simulink model "PowerGenSim_Attitude"  (R2024b)
settings: Solver=ode3  StartTime=0.0  StopTime=sat.T  FixedStep=10  MaxStep=113.53623125513354  RelTol=1e-3
values from neighbouring files (symbols this model uses):
  Re = 6378e03    (= 6378000)    [PowerGenSim_Params.m]
undefined symbols (not defined in the file or in its folder): sat
libraries: sharedtransform x4, vrlib x4, slpidlib x4, matrix_library x2, aerolibutil x1, sharedutil x1, aerolibsatdyn x1, simulink_extras x1
settings Model: Creator=Ameya  LastModifiedBy=Ameya

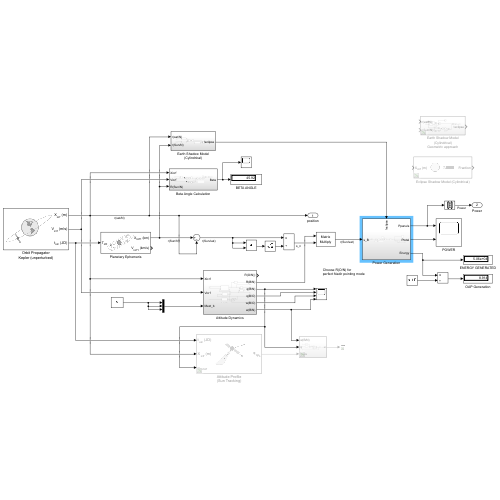
[thumbnail: Simulink's stored preview of the top-level diagram]
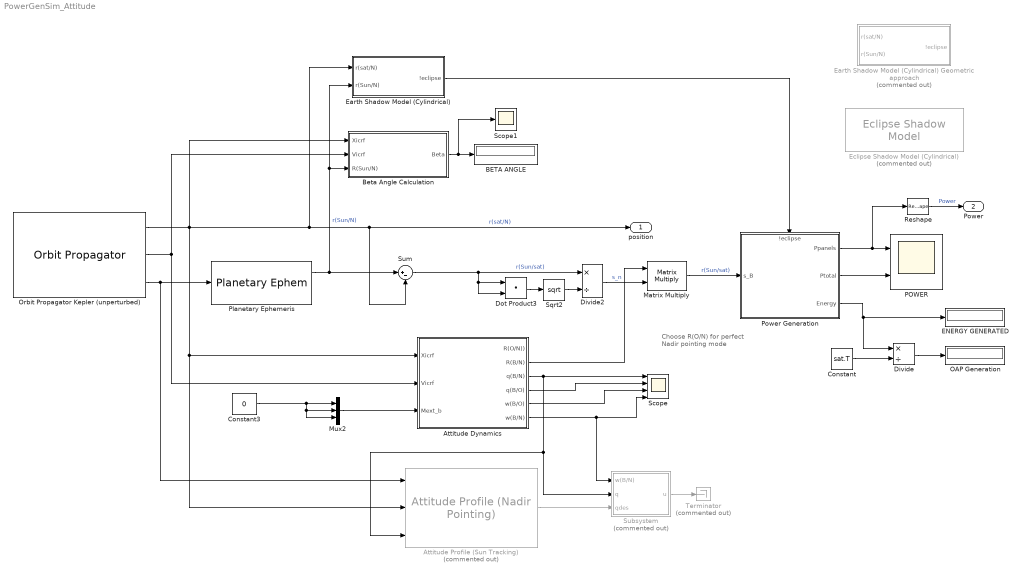
== system PowerGenSim_Attitude ==
  note: Choose R(O/N) for
      | perfect Nadir pointing mode
  Attitude Dynamics : Subsystem
  Attitude Profile (Sun Tracking) : aerolibsatdyn/Attitude Profile (Nadir Pointing)  Commented=on  outputError=on  outputFinalAttitude=off  portFrame=ICRF  pointingMode=Point at celestial body  celestialTarget=Sun  tunablePointing=off  primaryAlignmentSrc=Dialog  primaryAlignment=[0 0 1]  secondaryAlignmentSrc=Dialog  secondaryAlignment=[1 0 0]  constraintFrame=ICRF  primaryConstraintSrc=Dialog  primaryConstraint=[1 0 0]  secondaryConstraintSrc=Dialog  secondaryConstraint=[0 1 0]
      settings: LibrarySourceBlock=|
      | aerolibsatdyn/Attitude Profile
      | (Sun Tracking)
  BETA ANGLE : Display
  Beta Angle Calculation : Subsystem
  Constant : Constant  Value=sat.T
  Constant3 : Constant  Value=0
  Divide : Product  Inputs=*/
  Divide2 : Product  Inputs=*/
  Dot Product3 : DotProduct  OutDataTypeStr=Inherit: Inherit via internal rule
  ENERGY GENERATED : Display
  Earth Shadow Model (Cylindrical) : Subsystem
  Earth Shadow Model (Cylindrical) Geometric approach : Subsystem  Commented=on
  Eclipse Shadow Model (Cylindrical) : EclipseShadowModel  Commented=on  shadowModel=Cylindrical  startDate=initialTimeJD  includeMoon=off  useEphemerisDateRange=off
  Matrix Multiply : Product  Multiplication=Matrix(*)
  Mux2 : Mux  Inputs=3
  OAP Generation : Display
  Orbit Propagator Kepler (unperturbed) : OrbitPropagator  startDate=initialTimeJD  semiMajorAxis=sat.a  eccentricity=sat.e  inclination=sat.i  raan=sat.RAAN  argPeriapsis=sat.w  trueAnomaly=sat.f  inertialPosition=[3649700.0 3308200.0 -4676600.0]  inertialVelocity=[-2750.8 6666.4 2573.4]  fixedPosition=[-4142689.0 -2676864.7 -4669861.6]  fixedVelocity=[1452.7 -6720.7 2568.1]  customR=3396200  customMu=4.305e13  customJ2=1.0826269e-03  customOmega=4.06125949e-3
  POWER : Scope  NumInputPorts=2
  Planetary Ephemeris : PlanetaryEphem  target=Sun
  Power Generation : Subsystem
      settings: PortSchema="{\"entries\":[{\"content\":{\"sides\":[{\"content\":{\"connectorIds\":[\"In1\"]},\"type\":\"ConnectorPlacement.EquallySpacedRectSide\",\"uuid\":\"8d446733-69e8-48a0-ae35-006265559fdb\"},{\"content\":{\"connectorIds\":[\"Out1\",\"Out2\",\"Out3\"],\"side\":\"RIGHT\"},\"type\":\"ConnectorPlacement.EquallySpacedRectSide\",\"uuid\":\"081b3f49-1ee9-4aa1-bea1-61239cdc4507\"},{\"content\":{\"connectorIds\":[\"In2\"],\"side\":\"TOP\"},\"type\":\"ConnectorPlacement.EquallySpacedRectSide\",\"uuid\":\"b68fd0b1-c1d0-4a3a-b207-adf3131eec8b\"}]},\"type\":\"ConnectorPlacement.EquallySpacedConnector\",\"uuid\":\"c5f8928d-ef3b-4c68-b6c6-8ab80b1a820a\"}],\"packageUris\":[\"http://schema.mathworks.com/mf0/Connector/R2020b\"],\"version\":\"1.0\"}"
  Reshape : Reshape  OutputDimensionality=Column vector (2-D)
  Scope : Scope  NumInputPorts=4
  Scope1 : Scope
  Sqrt2 : Sqrt
  Subsystem : Subsystem  Commented=on
  Sum : Sum  Inputs=|+-
  Terminator : Terminator  Commented=on
  position : Outport
  Power : Outport  Port=2
  wires:
  Divide/1 -> OAP Generation/1
  Earth Shadow Model (Cylindrical)/1(!eclipse) -> Power Generation/2(!eclipse)
  Power Generation/1(Ppanels) -> Reshape/1, POWER/1
  Orbit Propagator Kepler (unperturbed)/3 -> Attitude Profile (Sun Tracking)/1, Planetary Ephemeris/1
  Planetary Ephemeris/1 -> Earth Shadow Model (Cylindrical)/2(r(Sun/N)), Beta Angle Calculation/3(R(Sun/N)), Sum/1  "r(Sun/N)"
  Reshape/1 -> Power/1  "Power"
  Power Generation/3(Energy) -> Divide/1, ENERGY GENERATED/1
  Constant/1 -> Divide/2
  Beta Angle Calculation/1(Beta) -> Scope1/1, BETA ANGLE/1
  Sqrt2/1 -> Divide2/2
  Power Generation/2(Ptotal) -> POWER/2
  Orbit Propagator Kepler (unperturbed)/2 -> Beta Angle Calculation/2(Vicrf), Attitude Dynamics/2(Vicrf)
  Divide2/1 -> Matrix Multiply/2  "s_n"
  Orbit Propagator Kepler (unperturbed)/1 -> Attitude Profile (Sun Tracking)/2, Attitude Dynamics/1(Xicrf), Beta Angle Calculation/1(Xicrf), Earth Shadow Model (Cylindrical)/1(r(sat/N)), position/1, Sum/2  "r(sat/N)"
  Dot Product3/1 -> Sqrt2/1
  Sum/1 -> Dot Product3/2, Dot Product3/1, Divide2/1  "r(Sun/sat)"
  Attitude Dynamics/2(R(B/N)) -> Matrix Multiply/1
  Constant3/1 -> Mux2/3, Mux2/2, Mux2/1
  Attitude Dynamics/3(q(B/N)) -> Subsystem/2(q), Attitude Profile (Sun Tracking)/3, Scope/1
  Attitude Dynamics/6(w(B/N)) -> Scope/4, Subsystem/1(w(B/N))
  Attitude Dynamics/4(q(B/O)) -> Scope/2
  Attitude Dynamics/5(w(B/O)) -> Scope/3
  Attitude Profile (Sun Tracking)/1 -> Subsystem/3(qdes)
  Subsystem/1(u) -> Terminator/1
  Mux2/1 -> Attitude Dynamics/3(Mext_b)
  Matrix Multiply/1 -> Power Generation/1(s_B)  "r(Sun/sat)"

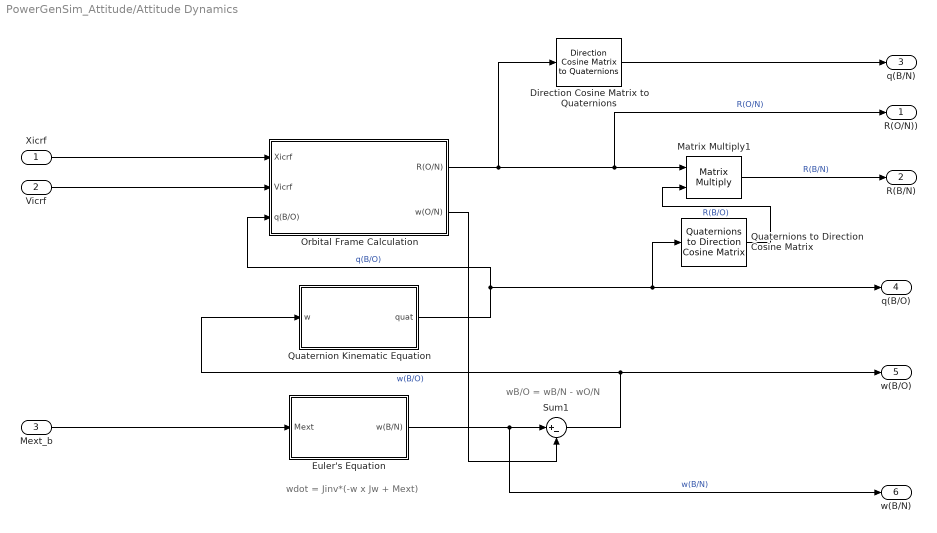
== system PowerGenSim_Attitude/Attitude Dynamics ==
  note: wdot = Jinv*(-w x Jw + Mext)
  note: wB/O = wB/N - wO/N
  Xicrf : Inport
  Vicrf : Inport  Port=2
  Mext_b : Inport  Port=3
  Direction Cosine Matrix to Quaternions : sharedtransform/Direction Cosine Matrix  to Quaternions  aMode=0  action=None  tolerance=eps(2)
      settings: LibrarySourceBlock=|
      | aerolibtransform2/Direction Cosine Matrix
      | to Quaternions
  Euler's Equation : Subsystem
  Matrix Multiply1 : Product  Multiplication=Matrix(*)
  Orbital Frame Calculation : Subsystem
  Quaternion Kinematic Equation : Subsystem
  Quaternions to Direction Cosine Matrix : sharedtransform/Quaternions to  Direction Cosine Matrix  aMode=aMode
      settings: LibrarySourceBlock=|
      | aerolibtransform2/Quaternions to
      | Direction Cosine Matrix
  Sum1 : Sum  Inputs=|+-
  R(O/N)) : Outport
  R(B/N) : Outport  Port=2
  q(B/N) : Outport  Port=3
  q(B/O) : Outport  Port=4
  w(B/O) : Outport  Port=5
  w(B/N) : Outport  Port=6
  wires:
  Quaternions to Direction Cosine Matrix/1 -> Matrix Multiply1/2  "R(B/O)"
  Euler's Equation/1(w(B/N)) -> w(B/N)/1, Sum1/1  "w(B/N)"
  Quaternion Kinematic Equation/1(quat) -> Orbital Frame Calculation/3(q(B/O)), q(B/O)/1, Quaternions to Direction Cosine Matrix/1  "q(B/O)"
  Orbital Frame Calculation/1(R(O/N)) -> Direction Cosine Matrix to Quaternions/1, R(O/N))/1, Matrix Multiply1/1  "R(O/N)"
  Orbital Frame Calculation/2(w(O/N)) -> Sum1/2
  Matrix Multiply1/1 -> R(B/N)/1  "R(B/N)"
  Sum1/1 -> w(B/O)/1, Quaternion Kinematic Equation/1(w)  "w(B/O)"
  Vicrf/1 -> Orbital Frame Calculation/2(Vicrf)
  Mext_b/1 -> Euler's Equation/1(Mext)
  Xicrf/1 -> Orbital Frame Calculation/1(Xicrf)
  Direction Cosine Matrix to Quaternions/1 -> q(B/N)/1

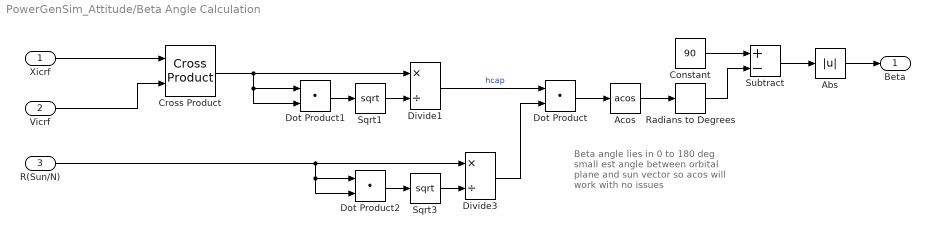
== system PowerGenSim_Attitude/Beta Angle Calculation ==
  note: Beta angle lies in 0 to 180 deg
      | small est angle between orbital plane and sun vector
      | so acos will work with no issues
  Xicrf : Inport
  Vicrf : Inport  Port=2
  R(Sun/N) : Inport  Port=3
  Abs : Abs  SaturateOnIntegerOverflow=off
  Acos : Trigonometry  Operator=acos
  Constant : Constant  Value=90
  Cross Product : matrix_library/Cross Product
  Divide1 : Product  Inputs=*/
  Divide3 : Product  Inputs=*/
  Dot Product : DotProduct  OutDataTypeStr=Inherit: Inherit via internal rule
  Dot Product1 : DotProduct  OutDataTypeStr=Inherit: Inherit via internal rule
  Dot Product2 : DotProduct  OutDataTypeStr=Inherit: Inherit via internal rule
  Radians to Degrees : simulink_extras/Transformations/Radians to Degrees
  Sqrt1 : Sqrt
  Sqrt3 : Sqrt
  Subtract : Sum  Inputs=+-
  Beta : Outport
  wires:
  Divide3/1 -> Dot Product/2
  Sqrt3/1 -> Divide3/2
  Dot Product/1 -> Acos/1
  Dot Product2/1 -> Sqrt3/1
  Cross Product/1 -> Dot Product1/1, Dot Product1/2, Divide1/1
  Acos/1 -> Radians to Degrees/1
  R(Sun/N)/1 -> Dot Product2/2, Dot Product2/1, Divide3/1
  Divide1/1 -> Dot Product/1  "hcap"
  Sqrt1/1 -> Divide1/2
  Dot Product1/1 -> Sqrt1/1
  Vicrf/1 -> Cross Product/2
  Radians to Degrees/1 -> Subtract/2
  Xicrf/1 -> Cross Product/1
  Constant/1 -> Subtract/1
  Subtract/1 -> Abs/1
  Abs/1 -> Beta/1

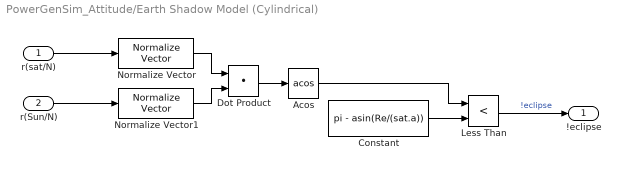
== system PowerGenSim_Attitude/Earth Shadow Model (Cylindrical) ==
  r(sat/N) : Inport
  r(Sun/N) : Inport  Port=2
  Acos : Trigonometry  Operator=acos
  Constant : Constant  Value=pi - asin(Re/(sat.a))
  Dot Product : DotProduct  OutDataTypeStr=Inherit: Inherit via internal rule
  Less Than : RelationalOperator  Operator=<  OutDataTypeStr=boolean  RndMeth=Simplest  InputSameDT=off
  Normalize Vector : vrlib/Utilities/Normalize Vector  maxzero=0
  Normalize Vector1 : vrlib/Utilities/Normalize Vector  maxzero=0
  !eclipse : Outport
  wires:
  Constant/1 -> Less Than/2
  r(sat/N)/1 -> Normalize Vector/1
  Less Than/1 -> !eclipse/1  "!eclipse"
  Normalize Vector/1 -> Dot Product/1
  Normalize Vector1/1 -> Dot Product/2
  Dot Product/1 -> Acos/1
  Acos/1 -> Less Than/1
  r(Sun/N)/1 -> Normalize Vector1/1

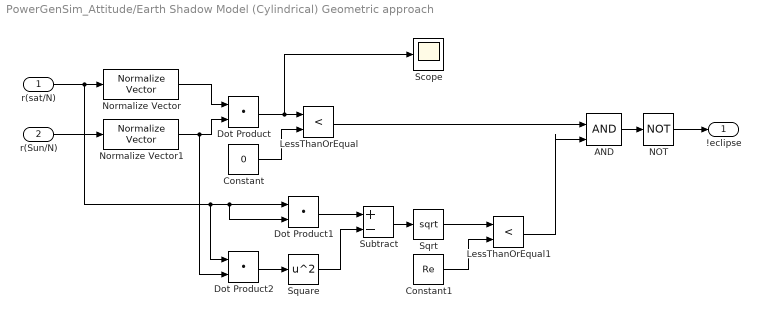
== system PowerGenSim_Attitude/Earth Shadow Model (Cylindrical) Geometric approach ==
  r(sat/N) : Inport
  r(Sun/N) : Inport  Port=2
  AND : Logic  IconShape=distinctive  AllPortsSameDT=off  OutDataTypeStr=boolean
  Constant : Constant  Value=0
  Constant1 : Constant  Value=Re
  Dot Product : DotProduct  OutDataTypeStr=Inherit: Inherit via internal rule
  Dot Product1 : DotProduct  OutDataTypeStr=Inherit: Inherit via internal rule
  Dot Product2 : DotProduct  OutDataTypeStr=Inherit: Inherit via internal rule
  LessThanOrEqual : RelationalOperator  Operator=<  OutDataTypeStr=boolean  RndMeth=Simplest  InputSameDT=off
  LessThanOrEqual1 : RelationalOperator  Operator=<  OutDataTypeStr=boolean  RndMeth=Simplest  InputSameDT=off
  NOT : Logic  Operator=NOT  IconShape=distinctive  AllPortsSameDT=off  OutDataTypeStr=boolean
  Normalize Vector : vrlib/Utilities/Normalize Vector  maxzero=0
  Normalize Vector1 : vrlib/Utilities/Normalize Vector  maxzero=0
  Scope : Scope
  Sqrt : Sqrt
  Square : Math  Operator=square
  Subtract : Sum  Inputs=+-
  !eclipse : Outport
  wires:
  r(sat/N)/1 -> Dot Product1/2, Dot Product1/1, Dot Product2/1, Normalize Vector/1
  Normalize Vector/1 -> Dot Product/1
  Normalize Vector1/1 -> Dot Product/2, Dot Product2/2
  Dot Product/1 -> Scope/1, LessThanOrEqual/1
  r(Sun/N)/1 -> Normalize Vector1/1
  Constant/1 -> LessThanOrEqual/2
  Dot Product1/1 -> Subtract/1
  Square/1 -> Subtract/2
  Subtract/1 -> Sqrt/1
  Sqrt/1 -> LessThanOrEqual1/1
  Constant1/1 -> LessThanOrEqual1/2
  LessThanOrEqual/1 -> AND/1
  LessThanOrEqual1/1 -> AND/2
  AND/1 -> NOT/1
  Dot Product2/1 -> Square/1
  NOT/1 -> !eclipse/1

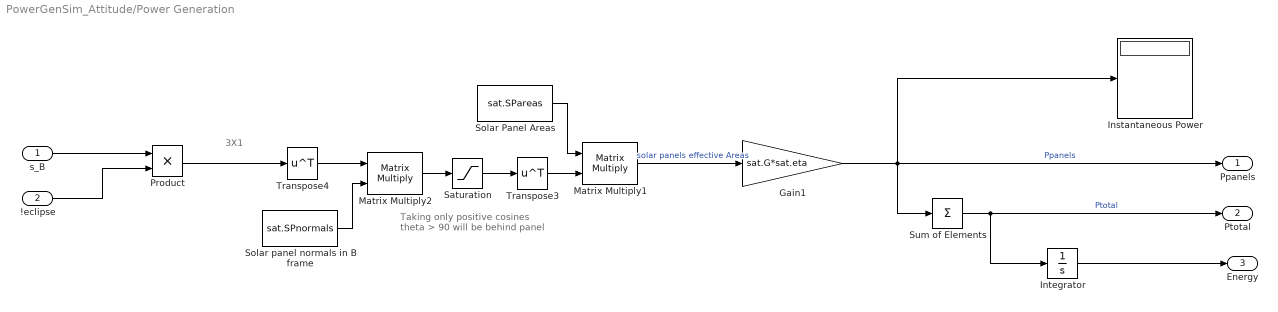
== system PowerGenSim_Attitude/Power Generation ==
  note: 3X1
  note: Taking only positive cosines
      | theta > 90 will be behind panel
  s_B : Inport
  !eclipse : Inport  Port=2
  Gain1 : Gain  Gain=sat.G*sat.eta
  Instantaneous Power : Display
  Integrator : Integrator
  Matrix Multiply1 : Product  Multiplication=Matrix(*)
  Matrix Multiply2 : Product  Multiplication=Matrix(*)
  Product : Product
  Saturation : Saturate  UpperLimit=inf  LowerLimit=0
  Solar Panel Areas : Constant  Value=sat.SPareas
  Solar panel normals in B frame : Constant  Value=sat.SPnormals
  Sum of Elements : Sum  Inputs=+
  Transpose3 : Math  Operator=transpose
  Transpose4 : Math  Operator=transpose
  Ppanels : Outport
  Ptotal : Outport  Port=2
  Energy : Outport  Port=3
  wires:
  Saturation/1 -> Transpose3/1
  Sum of Elements/1 -> Ptotal/1, Integrator/1  "Ptotal"
  Matrix Multiply1/1 -> Gain1/1  "solar panels effective Areas"
  Transpose3/1 -> Matrix Multiply1/2
  Gain1/1 -> Ppanels/1, Sum of Elements/1, Instantaneous Power/1  "Ppanels"
  Transpose4/1 -> Matrix Multiply2/1
  s_B/1 -> Product/1
  Solar panel normals in B frame/1 -> Matrix Multiply2/2
  Solar Panel Areas/1 -> Matrix Multiply1/1
  Matrix Multiply2/1 -> Saturation/1
  Integrator/1 -> Energy/1
  Product/1 -> Transpose4/1
  !eclipse/1 -> Product/2

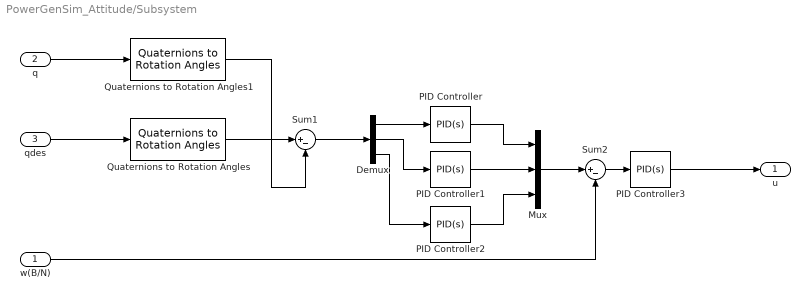
== system PowerGenSim_Attitude/Subsystem ==
  w(B/N) : Inport
  q : Inport  Port=2
  qdes : Inport  Port=3
  Demux : Demux  Outputs=3
  Mux : Mux  Inputs=3
  PID Controller{,1..3} (4 alike) : slpidlib/PID Controller  Controller=PID  Form=Parallel  TimeDomain=Continuous-time  UseExternalTs=off  SampleTime=-1  IntegratorMethod=Forward Euler  FilterMethod=Forward Euler  ControllerParametersSource=internal  P=1  I=1  UseKiTs=off  D=0  UseExternalDerivativeSource=off  N=100  UseFilter=on  TunerSelectOption=Transfer Function Based (PID Tuner App)  InitialConditionSource=internal  InitialConditionForIntegrator=0  InitialConditionForFilter=0  DifferentiatorICPrevScaledInput=0  ExternalReset=none  TrackingMode=off  Kt=1  LimitOutput=off  SatLimitsSource=internal  UpperSaturationLimit=inf  LowerSaturationLimit=-inf  LinearizeAsGain=on  AntiWindupMode=none  Kb=1  LimitIntegrator=off  UpperIntegratorSaturationLimit=inf  LowerIntegratorSaturationLimit=-inf  POutMin=[]  POutMax=[]  IOutMin=[]  IOutMax=[]  DOutMin=[]  DOutMax=[]  NOutMin=[]  NOutMax=[]  SumOutMin=[]  SumOutMax=[]  SaturationOutMin=[]  SaturationOutMax=[]  PParamMin=[]  PParamMax=[]  IParamMin=[]  IParamMax=[]  DParamMin=[]  DParamMax=[]  NParamMin=[]  NParamMax=[]  KbParamMin=[]  KbParamMax=[]  KtParamMin=[]  KtParamMax=[]  KbOutMin=[]  KbOutMax=[]  KtOutMin=[]  KtOutMax=[]  IntegratorOutMin=[]  IntegratorOutMax=[]  FilterOutMin=[]  FilterOutMax=[]  SumI1OutMin=[]  SumI1OutMax=[]  SumI2OutMin=[]  SumI2OutMax=[]  SumI3OutMin=[]  SumI3OutMax=[]  SumI4OutMin=[]  SumI4OutMax=[]  SumDOutMin=[]  SumDOutMax=[]  DifferentiatorOutMin=[]  DifferentiatorOutMax=[]  FilterDiffOutCoefMin=[]  FilterDiffOutCoefMax=[]  ReciprocalOutMin=[]  ReciprocalOutMax=[]  SumDenOutMin=[]  SumDenOutMax=[]  SumNumOutMin=[]  SumNumOutMax=[]  DivideOutMin=[]  DivideOutMax=[]  UdiffTsProdOutMin=[]  UdiffTsProdOutMax=[]  NTsProdOutMin=[]  NTsProdOutMax=[]  UintegralTsProdOutMin=[]  UintegralTsProdOutMax=[]  UngainTsProdOutMin=[]  UngainTsProdOutMax=[]  ClampingZeroOutDataTypeStr=Inherit: Inherit via back propagation  ClampingZeroOutMin=[]  ClampingZeroOutMax=[]  FilterDenConstantOutDataTypeStr=Inherit: Inherit via back propagation  FilterDenConstantOutMin=[]  FilterDenConstantOutMax=[]  PCopyOutDataTypeStr=Inherit: Inherit via back propagation  PCopyOutMin=[]  PCopyOutMax=[]  NCopyOutDataTypeStr=Inherit: Inherit via back propagation  NCopyOutMin=[]  NCopyOutMax=[]  IntegratorContinuousStateAttributes=''  IntegratorStateMustResolveToSignalObject=off  IntegratorRTWStateStorageClass=Auto  FilterContinuousStateAttributes=''  FilterStateMustResolveToSignalObject=off  FilterRTWStateStorageClass=Auto  ParallelPVariant=InternalParameters  IdealPVariant=Disabled  IVariant=InternalParameters  DVariant=InternalParameters  IntegratorVariant=Continuous  SatVariant=Disabled  AWVariant=Passthrough  PCopyVariant=Disabled  TRVariant=Disabled  FdbkBlocksVariant=Forward  IdealPFdbkVariant=Disabled  SatFdbkVariant=Disabled  DerivativeFilterVariant=ContFilter  NVariant=InternalParameters  NCopyVariant=Disabled  FilterICVariant=InternalICsFilter  IntegratorICVariant=InternalICs  ExternalResetVariant=Disabled  TRSumVariant=Passthrough  SumFdbkVariant=Disabled  SumVariant=Sum_PID  TsampFilterVariant=InternalTs  TsampNgainVariant=Passthrough  TsampIntegralVariant=Disabled_SignalSpec  ExternalSaturationOutDataTypeStr=Inherit: Same as second input  DerivativeSourceVariant=ErrorSignal  PreIntVariant=InternalPreInt
  Quaternions to Rotation Angles : sharedtransform/Quaternions to Rotation Angles  rotationOrder=ZYX  aMode=aMode
  Quaternions to Rotation Angles1 : sharedtransform/Quaternions to Rotation Angles  rotationOrder=ZYX  aMode=aMode
  Sum1 : Sum  Inputs=|+-
  Sum2 : Sum  Inputs=|+-
  u : Outport
  wires:
  PID Controller1/1 -> Mux/2
  Quaternions to Rotation Angles1/1 -> Sum1/2
  Demux/3 -> PID Controller2/1
  Quaternions to Rotation Angles/1 -> Sum1/1
  PID Controller2/1 -> Mux/3
  Sum2/1 -> PID Controller3/1
  Demux/2 -> PID Controller1/1
  PID Controller/1 -> Mux/1
  Sum1/1 -> Demux/1
  Demux/1 -> PID Controller/1
  w(B/N)/1 -> Sum2/2
  Mux/1 -> Sum2/1
  q/1 -> Quaternions to Rotation Angles1/1
  qdes/1 -> Quaternions to Rotation Angles/1
  PID Controller3/1 -> u/1

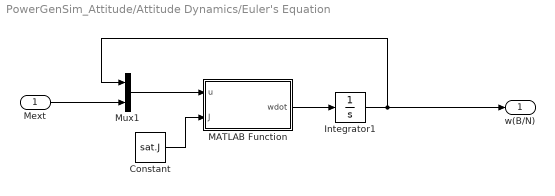
== system PowerGenSim_Attitude/Attitude Dynamics/Euler's Equation ==
  Mext : Inport
  Constant : Constant  Value=sat.J
  Integrator1 : Integrator  InitialCondition=sat.omegaBN
  MATLAB Function : MATLAB Function  TreatAsAtomicUnit=on
  Mux1 : Mux  Inputs=2
  w(B/N) : Outport
  wires:
  Mext/1 -> Mux1/2
  MATLAB Function/1(wdot) -> Integrator1/1
  Integrator1/1 -> Mux1/1, w(B/N)/1
  Mux1/1 -> MATLAB Function/1(u)
  Constant/1 -> MATLAB Function/2(J)

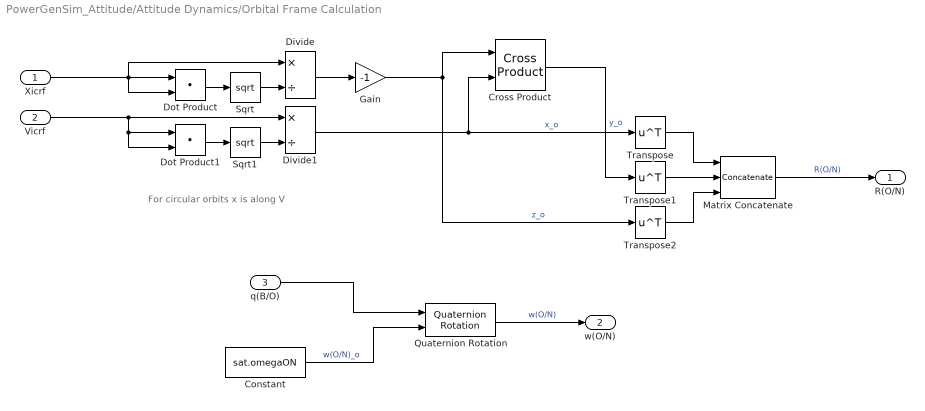
== system PowerGenSim_Attitude/Attitude Dynamics/Orbital Frame Calculation ==
  note: For circular orbits x is along V
  Xicrf : Inport
  Vicrf : Inport  Port=2
  q(B/O) : Inport  Port=3
  Constant : Constant  Value=sat.omegaON
  Cross Product : matrix_library/Cross Product
  Divide : Product  Inputs=*/
  Divide1 : Product  Inputs=*/
  Dot Product : DotProduct  OutDataTypeStr=Inherit: Inherit via internal rule
  Dot Product1 : DotProduct  OutDataTypeStr=Inherit: Inherit via internal rule
  Gain : Gain  Gain=-1
  Matrix Concatenate : Concatenate  NumInputs=3  Mode=Multidimensional array
  Quaternion Rotation : aerolibutil/Quaternion Rotation
  Sqrt : Sqrt
  Sqrt1 : Sqrt
  Transpose : Math  Operator=transpose
  Transpose1 : Math  Operator=transpose
  Transpose2 : Math  Operator=transpose
  R(O/N) : Outport
  w(O/N) : Outport  Port=2
  wires:
  Transpose2/1 -> Matrix Concatenate/3
  Dot Product/1 -> Sqrt/1
  Vicrf/1 -> Dot Product1/1, Dot Product1/2, Divide1/1
  Divide1/1 -> Transpose/1, Cross Product/2  "x_o"
  Xicrf/1 -> Divide/1, Dot Product/1, Dot Product/2
  Transpose/1 -> Matrix Concatenate/1
  Cross Product/1 -> Transpose1/1  "y_o"
  Divide/1 -> Gain/1
  Sqrt/1 -> Divide/2
  Sqrt1/1 -> Divide1/2
  Dot Product1/1 -> Sqrt1/1
  Transpose1/1 -> Matrix Concatenate/2
  Matrix Concatenate/1 -> R(O/N)/1  "R(O/N)"
  q(B/O)/1 -> Quaternion Rotation/1
  Constant/1 -> Quaternion Rotation/2  "w(O/N)_o"
  Quaternion Rotation/1 -> w(O/N)/1  "w(O/N)"
  Gain/1 -> Transpose2/1, Cross Product/1  "z_o"

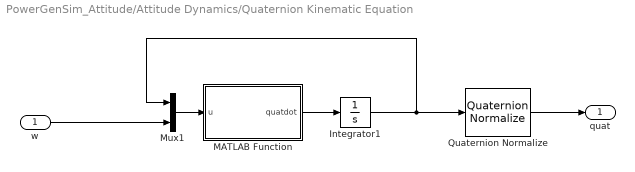
== system PowerGenSim_Attitude/Attitude Dynamics/Quaternion Kinematic Equation ==
  w : Inport
  Integrator1 : Integrator  InitialCondition=sat.quat
  MATLAB Function : MATLAB Function  TreatAsAtomicUnit=on
  Mux1 : Mux  Inputs=2
  Quaternion Normalize : sharedutil/Quaternion Normalize  aMode=aMode
  quat : Outport
  wires:
  Mux1/1 -> MATLAB Function/1(u)
  Integrator1/1 -> Quaternion Normalize/1, Mux1/1
  MATLAB Function/1(quatdot) -> Integrator1/1
  w/1 -> Mux1/2
  Quaternion Normalize/1 -> quat/1

== matlab function PowerGenSim_Attitude/Attitude Dynamics/Euler's Equation/MATLAB Function ==
  data: u input; wdot output; J input
function wdot = EulersEOM(u,J)
    w = u(1:3);
    m = u(4:6);
    wdot = J\(-cross(w,(J*w))+m);
end

== matlab function PowerGenSim_Attitude/Attitude Dynamics/Quaternion Kinematic Equation/MATLAB Function ==
  data: u input; quatdot output
function quatdot = quatKinematics(u)
    quat = u(1:4);
    p = u(5);
    q = u(6);
    r = u(7);
    quatdot = 0.5*[0,-p,-q,-r;
                p,0,r,-q;
                q,-r,0,p;
                r,q,-p,0]*quat;
end
